simulink subsystem "LOGGING"  (R2025b)
settings: Solver=VariableStepAuto  StartTime=0.0  StopTime=10.0  RelTol=1e-3
settings Model: Creator=antoniohernandez-rodiciomateos  LastModifiedBy=antoniohernandez-rodiciomateos

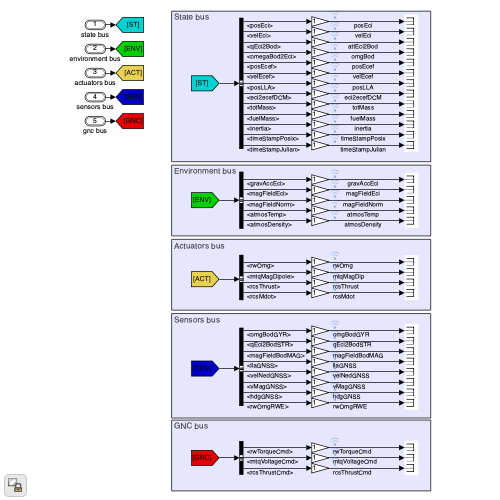
[thumbnail: Simulink's stored preview of the top-level diagram]
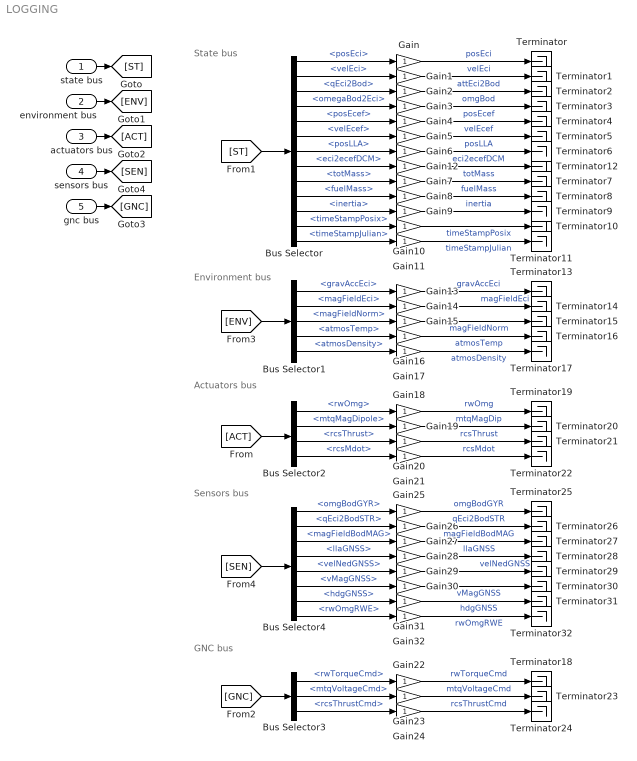
== system LOGGING ==
  note: State bus
  note: Environment bus
  note: Actuators bus
  note: GNC bus
  note: Sensors bus
  state bus : Inport  OutDataTypeStr=Bus: state_bus
  environment bus : Inport  Port=2  OutDataTypeStr=Bus: environment_bus
  actuators bus : Inport  Port=3  OutDataTypeStr=Bus: actuators_bus
  sensors bus : Inport  Port=4  OutDataTypeStr=Bus: sensors_bus
  gnc bus : Inport  Port=5  OutDataTypeStr=Bus: gnc_bus
  Bus Selector : BusSelector  OutputSignals=posEci,velEci,qEci2Bod,omegaBod2Eci,posEcef,velEcef,posLLA,eci2ecefDCM,totMass,fuelMass,inertia,timeStampPosix,timeStampJulian
  Bus Selector1 : BusSelector  OutputSignals=gravAccEci,magFieldEci,magFieldNorm,atmosTemp,atmosDensity
  Bus Selector2 : BusSelector  OutputSignals=rwOmg,mtqMagDipole,rcsThrust,rcsMdot
  Bus Selector3 : BusSelector  OutputSignals=rwTorqueCmd,mtqVoltageCmd,rcsThrustCmd
  Bus Selector4 : BusSelector  OutputSignals=omgBodGYR,qEci2BodSTR,magFieldBodMAG,llaGNSS,velNedGNSS,vMagGNSS,hdgGNSS,rwOmgRWE
  Gain{,1..32} (33 alike) : Gain
  Terminator{,1..32} (33 alike) : Terminator
  wires:
  state bus/1 -> [ST]
  [ST] -> Bus Selector/1
  Bus Selector/1 -> Gain/1  "<posEci>"
  Gain/1 -> Terminator/1  "posEci"
  Bus Selector/2 -> Gain1/1  "<velEci>"
  Gain1/1 -> Terminator1/1  "velEci"
  Gain3/1 -> Terminator3/1  "omgBod"
  Gain2/1 -> Terminator2/1  "attEci2Bod"
  Bus Selector/3 -> Gain2/1  "<qEci2Bod>"
  Bus Selector/4 -> Gain3/1  "<omegaBod2Eci>"
  Gain6/1 -> Terminator6/1  "posLLA"
  Gain7/1 -> Terminator7/1  "totMass"
  Gain5/1 -> Terminator5/1  "velEcef"
  Gain4/1 -> Terminator4/1  "posEcef"
  Bus Selector/5 -> Gain4/1  "<posEcef>"
  Bus Selector/6 -> Gain5/1  "<velEcef>"
  Bus Selector/7 -> Gain6/1  "<posLLA>"
  Bus Selector/9 -> Gain7/1  "<totMass>"
  Gain10/1 -> Terminator10/1  "timeStampPosix"
  Gain9/1 -> Terminator9/1  "inertia"
  Gain8/1 -> Terminator8/1  "fuelMass"
  Gain11/1 -> Terminator11/1  "timeStampJulian"
  Bus Selector/10 -> Gain8/1  "<fuelMass>"
  Bus Selector/11 -> Gain9/1  "<inertia>"
  Bus Selector/12 -> Gain10/1  "<timeStampPosix>"
  Bus Selector/13 -> Gain11/1  "<timeStampJulian>"
  Bus Selector/8 -> Gain12/1  "<eci2ecefDCM>"
  Gain12/1 -> Terminator12/1  "eci2ecefDCM"
  environment bus/1 -> [ENV]
  [ENV] -> Bus Selector1/1
  Bus Selector1/1 -> Gain13/1  "<gravAccEci>"
  Bus Selector1/2 -> Gain14/1  "<magFieldEci>"
  Bus Selector1/3 -> Gain15/1  "<magFieldNorm>"
  Bus Selector1/4 -> Gain16/1  "<atmosTemp>"
  Bus Selector1/5 -> Gain17/1  "<atmosDensity>"
  Gain13/1 -> Terminator13/1  "gravAccEci"
  Gain14/1 -> Terminator14/1  "magFieldEci"
  Gain15/1 -> Terminator15/1  "magFieldNorm"
  Gain16/1 -> Terminator16/1  "atmosTemp"
  Gain17/1 -> Terminator17/1  "atmosDensity"
  actuators bus/1 -> [ACT]
  gnc bus/1 -> [GNC]
  [ACT] -> Bus Selector2/1
  Bus Selector2/1 -> Gain18/1  "<rwOmg>"
  Bus Selector2/2 -> Gain19/1  "<mtqMagDipole>"
  Bus Selector2/3 -> Gain20/1  "<rcsThrust>"
  Bus Selector2/4 -> Gain21/1  "<rcsMdot>"
  Gain18/1 -> Terminator19/1  "rwOmg"
  Gain19/1 -> Terminator20/1  "mtqMagDip"
  Gain20/1 -> Terminator21/1  "rcsThrust"
  Gain21/1 -> Terminator22/1  "rcsMdot"
  [GNC] -> Bus Selector3/1
  Gain23/1 -> Terminator23/1  "mtqVoltageCmd"
  Gain22/1 -> Terminator18/1  "rwTorqueCmd"
  Gain24/1 -> Terminator24/1  "rcsThrustCmd"
  Bus Selector3/1 -> Gain22/1  "<rwTorqueCmd>"
  Bus Selector3/2 -> Gain23/1  "<mtqVoltageCmd>"
  Bus Selector3/3 -> Gain24/1  "<rcsThrustCmd>"
  sensors bus/1 -> [SEN]
  Gain25/1 -> Terminator25/1  "omgBodGYR"
  Gain26/1 -> Terminator26/1  "qEci2BodSTR"
  Gain27/1 -> Terminator27/1  "magFieldBodMAG"
  Gain28/1 -> Terminator28/1  "llaGNSS"
  [SEN] -> Bus Selector4/1
  Bus Selector4/1 -> Gain25/1  "<omgBodGYR>"
  Bus Selector4/2 -> Gain26/1  "<qEci2BodSTR>"
  Bus Selector4/3 -> Gain27/1  "<magFieldBodMAG>"
  Bus Selector4/4 -> Gain28/1  "<llaGNSS>"
  Gain30/1 -> Terminator30/1  "vMagGNSS"
  Gain29/1 -> Terminator29/1  "velNedGNSS"
  Gain31/1 -> Terminator31/1  "hdgGNSS"
  Bus Selector4/5 -> Gain29/1  "<velNedGNSS>"
  Bus Selector4/6 -> Gain30/1  "<vMagGNSS>"
  Bus Selector4/7 -> Gain31/1  "<hdgGNSS>"
  Gain32/1 -> Terminator32/1  "rwOmgRWE"
  Bus Selector4/8 -> Gain32/1  "<rwOmgRWE>"
